simulink model "Robot_smlnk"  (Simulink 7.4)
settings: Solver=ode45  StartTime=0.0  StopTime=60  FixedStep=0.00005  MaxStep=0.01  RelTol=1e-6
undefined symbols (not defined in the file or in its folder): contr_name, sfunxy, uini, xini
settings Model: Creator=manuelmazo  LastModifiedBy=p261584  ExtModeAutoUpdateStatusClock=off
settings OptimizationCC: InitFltsAndDblsToZero=on
settings DebuggingCC: SaveWithParameterizedLinksMsg=none
settings GRTTargetCC: TargetFcnLib=ansi_tfl_tmw.mat

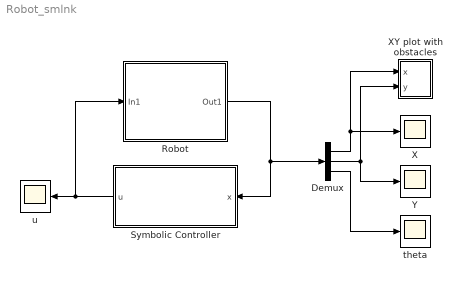
== system Robot_smlnk ==
  Demux : Demux  Outputs=3
  Robot : Subsystem
  "Symbolic Controller " : Subsystem  mask{contr_name=contr_name, uini=uini}
      mask prompts: contr_name "Controller Name"; uini "Initial Controller State"
      mask init:
      | load(strcat(contr_name,'_symb'), 'params_symb');
  X : Scope
      settings: YMin=19  YMax=20
  XY plot with obstacles : Subsystem  AncestorBlock=simulink/Sinks/XY Graph  LoadFcn=sfunxy([],[],[],'LoadBlock')  StartFcn=sfunxy([],[],[],'Start')  StopFcn=sfunxy([],[],[],'Stop')  TreatAsAtomicUnit=on  SimViewingDevice=on  mask(XY scope.){xmin=1, xmax=5, ymin=1, ymax=5, st=-1}
      mask prompts: xmin "x-min:"; xmax "x-max:"; ymin "y-min:"; ymax "y-max:"; st "Sample time:"
      mask help: Plots second input (Y) against first input (X) at each time step to create an X-Y plot. Ignores data outside the ranges specified by x-min, x-max, y-min, y-max.
      settings: CopyFcn=sfunxy([],[],[],'CopyBlock')  DeleteFcn=sfunxy([],[],[],'DeleteBlock')  NameChangeFcn=sfunxy([],[],[],'NameChange')
      mask Help: This block can be used to explore limit cycles. Look at the m-file sfunxy.m to see how it works.
      mask Display: plot([.05 .95 .95 .05 .05],[.45 .45 .95 .95 .45], 0.5+cos(0:0.1:2*pi)*0.3,0.7+sin(0:0.1:2*pi)*0.2)
  Y : Scope
      settings: YMin=-3  YMax=3  SaveName=ScopeData2
  theta : Scope
      settings: YMin=-3  YMax=3  SaveName=ScopeData4
  u : Scope
      settings: YMin=-1  YMax=1  SaveName=ScopeData3
  wires:
  Robot/1(Out1) -> Demux/1, "Symbolic Controller "/1(x)
  Demux/1 -> X/1, XY plot with obstacles/1(x)
  Demux/2 -> Y/1, XY plot with obstacles/2(y)
  "Symbolic Controller "/1(u) -> Robot/1(In1), u/1
  Demux/3 -> theta/1

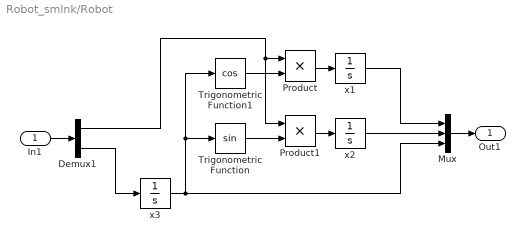
== system Robot_smlnk/Robot ==
  In1 : Inport  OutDataType=sfix(16)  OutScaling=2^0
  Demux1 : Demux  Outputs=2
  Mux : Mux  Inputs=3
  Product : Product  OutDataType=sfix(16)  OutScaling=2^0  RndMeth=Zero
  Product1 : Product  OutDataType=sfix(16)  OutScaling=2^0  RndMeth=Zero
  Trigonometric Function : Trigonometry
  Trigonometric Function1 : Trigonometry  Operator=cos
  x1 : Integrator  InitialCondition=xini(1)
  x2 : Integrator  InitialCondition=xini(2)
  x3 : Integrator  InitialCondition=xini(3)
  Out1 : Outport  OutDataType=sfix(16)  OutScaling=2^0
  wires:
  Demux1/2 -> x3/1
  x3/1 -> Trigonometric Function1/1, Trigonometric Function/1, Mux/3
  Trigonometric Function/1 -> Product1/2
  Trigonometric Function1/1 -> Product/2
  Demux1/1 -> Product/1, Product1/1
  Product/1 -> x1/1
  Product1/1 -> x2/1
  x1/1 -> Mux/1
  x2/1 -> Mux/2
  Mux/1 -> Out1/1
  In1/1 -> Demux1/1

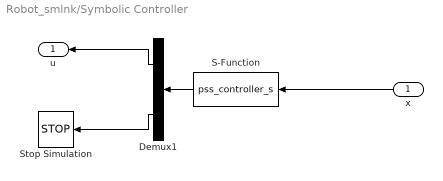
== system Robot_smlnk/Symbolic Controller  ==
  x : Inport  OutDataType=sfix(16)  OutScaling=2^0
  Demux1 : Demux  Outputs=2
  S-Function : S-Function  FunctionName=pss_controller_s  Parameters=params_symb, contr_name, uini  EnableBusSupport=off
  Stop Simulation : Stop
  u : Outport  OutDataType=sfix(16)  OutScaling=2^0
  wires:
  S-Function/1 -> Demux1/1
  x/1 -> S-Function/1
  Demux1/1 -> u/1
  Demux1/2 -> Stop Simulation/1

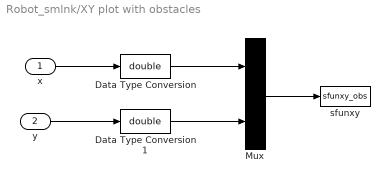
== system Robot_smlnk/XY plot with obstacles ==
  x : Inport  OutDataType=sfix(16)  OutScaling=2^0
  y : Inport  Port=2  OutDataType=sfix(16)  OutScaling=2^0
  Data Type Conversion : DataTypeConversion  OutDataTypeMode=double  OutDataType=sfix(16)  OutScaling=2^0  OutDataTypeStr=double
  Data Type Conversion1 : DataTypeConversion  OutDataTypeMode=double  OutDataType=sfix(16)  OutScaling=2^0  OutDataTypeStr=double
  Mux : Mux  Inputs=2
  sfunxy : S-Function  FunctionName=sfunxy_obs  Parameters=[xmin xmax ymin ymax], st  EnableBusSupport=off
  wires:
  Data Type Conversion1/1 -> Mux/2
  Data Type Conversion/1 -> Mux/1
  y/1 -> Data Type Conversion1/1
  x/1 -> Data Type Conversion/1
  Mux/1 -> sfunxy/1
